simulink model "PSK_2"  (R2017b)
settings: Solver=ode45  StartTime=0.0  StopTime=10  MaxStep=0.01  MinStep=0.00001  RelTol=1e-3
libraries: commchan3 x1, dsparch4 x1
settings Model: Creator=ayadd  LastModifiedBy=ayadd
settings SolverCC: ShapePreserveControl=EnableAll  ZeroCrossAlgorithm=Adaptive

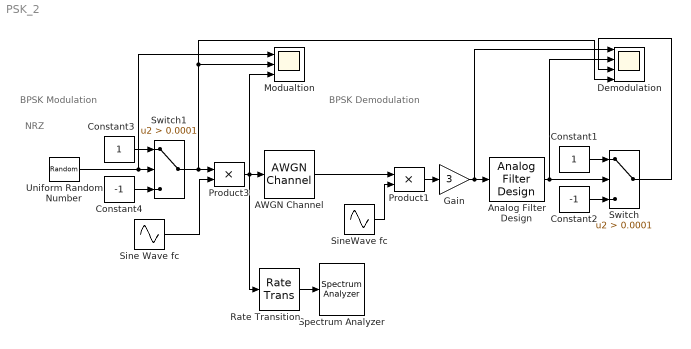
== system PSK_2 ==
  note: NRZ
  note: BPSK Demodulation
  note: BPSK Modulation
  AWGN Channel : commchan3/AWGN Channel  InputProcessing=Columns as channels (frame based)  seed=67  noiseMode="Signal to noise ratio  (SNR)"  EbNodB=10  EsNodB=10  SNRdB=30  bitsPerSym=1  Ps=1  Tsym=0.01  variance=1
  Analog Filter Design : dsparch4/Analog Filter Design  method=Butterworth  filttype=Lowpass  N=8  Wlo=10*2*pi  Whi=80  Rp=2  Rs=40
  Constant1 : Constant
  Constant2 : Constant  Value=-1
  Constant3 : Constant
  Constant4 : Constant  Value=-1
  Demodulation : Scope  NumInputPorts=4
  Gain : Gain  Gain=3
  Modualtion : Scope  NumInputPorts=3
  Product1 : Product  SaturateOnIntegerOverflow=on  InputSameDT=on  OutDataTypeStr=Inherit: Same as first input
  Product3 : Product  OutDataTypeStr=double  SaturateOnIntegerOverflow=on  InputSameDT=on
  Rate Transition : RateTransition  OutPortSampleTime=0.01
  Sine Wave fc : Sin  Frequency=4*2*pi  SampleTime=0
  SineWave fc : Sin  Frequency=4*2*pi  SampleTime=0
  Spectrum Analyzer : SpectrumAnalyzer
  Switch : Switch  Criteria=u2 > Threshold  Threshold=0.0001  RndMeth=Round  SaturateOnIntegerOverflow=on  InputSameDT=on
  Switch1 : Switch  Criteria=u2 > Threshold  Threshold=0.0001  RndMeth=Round  SaturateOnIntegerOverflow=on  InputSameDT=on
  Uniform Random Number : UniformRandomNumber  SampleTime=1
  wires:
  Uniform Random Number/1 -> Switch1/2, Modualtion/1
  Product1/1 -> Gain/1
  Analog Filter Design/1 -> Demodulation/2, Switch/2
  Gain/1 -> Demodulation/1, Analog Filter Design/1
  SineWave fc/1 -> Product1/2
  Sine Wave fc/1 -> Product3/2
  Switch1/1 -> Demodulation/4, Modualtion/2, Product3/1
  AWGN Channel/1 -> Product1/1
  Product3/1 -> Rate Transition/1, Modualtion/3, AWGN Channel/1
  Rate Transition/1 -> Spectrum Analyzer/1
  Constant1/1 -> Switch/1
  Constant2/1 -> Switch/3
  Switch/1 -> Demodulation/3
  Constant4/1 -> Switch1/3
  Constant3/1 -> Switch1/1
